simulink model "j3s"  (R2023b)
settings: Solver=VariableStepAuto  StartTime=0.0  StopTime=200  RelTol=1e-3
settings Model: Creator=asus  LastModifiedBy=asus

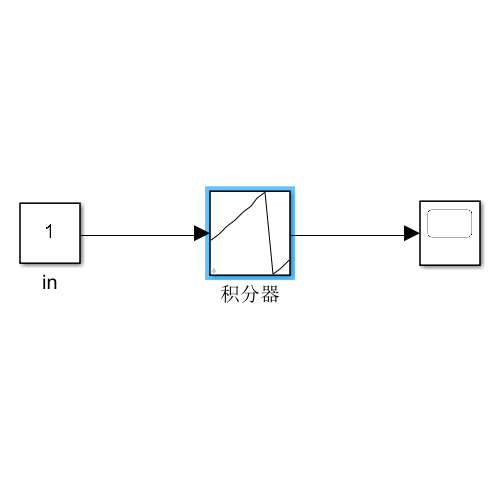
[thumbnail: Simulink's stored preview of the top-level diagram]
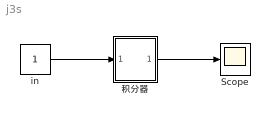
== system j3s ==
  Scope : Scope
  in : Constant
  积分器 : Subsystem  mask{chushizhi=-50, yuzhi=20, chongzhizhi=-100}
      mask prompts: chushizhi "初始条件"; yuzhi "输出阈值"; chongzhizhi "重置值"
      mask DialogControl ParameterGroupVar Prompt: 参数
      mask Display: plot([0 10 20 30 40 50 60 70 80 90 100], [-50 -40 -30 -20 -10 0 10 20 -100 -90 -80]);
  wires:
  in/1 -> 积分器/1(In2)
  积分器/1(Out1) -> Scope/1

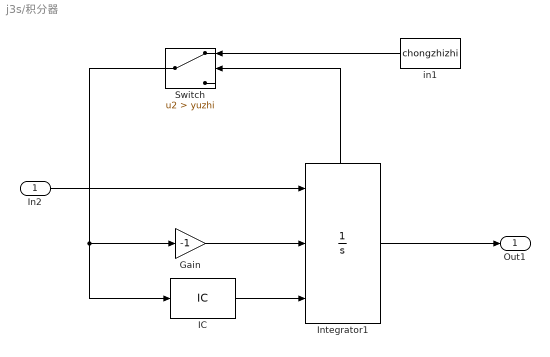
== system j3s/积分器 ==
  In2 : Inport
  Gain : Gain  Gain=-1
  IC : InitialCondition  Value=chushizhi
  Integrator1 : Integrator  ExternalReset=rising  InitialConditionSource=external  ShowStatePort=on
  Switch : Switch  Criteria=u2 > Threshold  Threshold=yuzhi  SaturateOnIntegerOverflow=off  InputSameDT=off
  in1 : Constant  Value=chongzhizhi
  Out1 : Outport
  wires:
  Integrator1/1 -> Out1/1
  Switch/1 -> Gain/1, IC/1
  IC/1 -> Integrator1/3
  in1/1 -> Switch/1
  In2/1 -> Integrator1/1
  Integrator1/State -> Switch/2
  Gain/1 -> Integrator1/2
